simulink model "simulation"  (R2014a)
settings: Solver=ode45  StartTime=0.0  StopTime=10.0  RelTol=1e-3
settings Model: Creator=flp  LastModifiedBy=flp

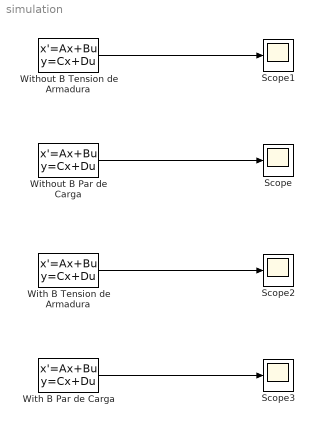
== system simulation ==
  Scope{,1..3} (4 alike) : Scope
      Scope2 settings: SaveName=ScopeData2
      Scope3 settings: SaveName=ScopeData3
  "With B Par de Carga " : StateSpace  A=[-0.0333 -7.9561 ; -0.1814 0]  B=[2.19298 0; 0 -0.05]  C=[0 1]  D=[0 0]  X0=[823 ; 1000]
  "With B Tension de Armadura " : StateSpace  A=[-0.0333 -7.9561 ; -0.1814 0]  B=[2.19298 0; 0 -0.05]  C=[1 0]  D=[0 0]  X0=[823 ; 1000]
  "Without B Par de Carga " : StateSpace  A=[-0.0333 -7.9561 ; -0.1814 0]  B="[0  0; 0 0]"  C=[0 1]  D=[0 0]  X0=[823 ; 1000]
  Without B Tension de Armadura : StateSpace  A=[-0.0333 -7.9561 ; -0.1814 0]  B="[0  0; 0 0]"  C=[1 0]  D=[0 0]  X0=[823 ; 1000]
  wires:
  "Without B Par de Carga "/1 -> Scope/1
  Without B Tension de Armadura/1 -> Scope1/1
  "With B Tension de Armadura "/1 -> Scope2/1
  "With B Par de Carga "/1 -> Scope3/1
